simulink library "Gait_Selector"  (R2024a)
settings: Solver=VariableStepAuto  StartTime=0.0  StopTime=10.0  RelTol=1e-3
undefined symbols (not defined in the file): Length_torso, sampleTime, transferFunVal, Width_torso
libraries: simulink_extras x12, stand_still_Gait x1, trot_Gait x1, turn_left_Gait x1, turn_right_Gait x1, walk_back_Gait x1, walk_Gait x1, walk_left_Gait x1, walk_right_Gait x1
(part 2 of 2)

== system Gait_Selector/Gait Selector/Trot Gait - Drive Function/right Back Hip gait/If Action Subsystem ==
  In1 : Inport
  tdur : Inport  Port=2
  Add : Sum  Inputs=+-
  Constant : Constant  Value=1.5 * pi
  Divide : Product  Inputs=*/
  Gain1 : Gain  Gain=2/3
  Gain4 : Gain  Gain=2*pi
  Sin : Trigonometry
  Out1 : Outport
  wires:
  In1/1 -> Gain4/1
  Constant/1 -> Add/2
  Add/1 -> Gain1/1
  Gain1/1 -> Sin/1
  Sin/1 -> Out1/1
  Gain4/1 -> Divide/1
  tdur/1 -> Divide/2
  Divide/1 -> Add/1

== system Gait_Selector/Gait Selector/Trot Gait - Drive Function/right Back Hip gait/If Action Subsystem1 ==
  In1 : Inport
  tdur : Inport  Port=2
  Add : Sum  Inputs=+-
  Constant : Constant  Value=1.0 * pi
  Divide : Product  Inputs=*/
  Gain1 : Gain  Gain=2
  Gain4 : Gain  Gain=2*pi
  Sin : Trigonometry
  Out1 : Outport
  wires:
  Sin/1 -> Out1/1
  In1/1 -> Gain4/1
  Add/1 -> Gain1/1
  Constant/1 -> Add/2
  Gain1/1 -> Sin/1
  Gain4/1 -> Divide/1
  Divide/1 -> Add/1
  tdur/1 -> Divide/2

== system Gait_Selector/Gait Selector/Trot Gait - Drive Function/right Back Hip gait/If Action Subsystem2 ==
  In1 : Inport
  tdur : Inport  Port=2
  Add : Sum  Inputs=+-
  Constant : Constant  Value=1.25 * pi
  Divide : Product  Inputs=*/
  Gain1 : Gain  Gain=2/3
  Gain4 : Gain  Gain=2*pi
  Sin : Trigonometry  Operator=cos
  Out1 : Outport
  wires:
  Sin/1 -> Out1/1
  In1/1 -> Gain4/1
  Add/1 -> Gain1/1
  Constant/1 -> Add/2
  Gain1/1 -> Sin/1
  Gain4/1 -> Divide/1
  Divide/1 -> Add/1
  tdur/1 -> Divide/2

== system Gait_Selector/Gait Selector/Trot Gait - Drive Function/right Back Knee gait/If Action Subsystem4 ==
  In1 : Inport
  tdur : Inport  Port=2
  Add : Sum  Inputs=+-
  Constant : Constant  Value=0.75 * pi
  Divide : Product  Inputs=*/
  Gain1 : Gain  Gain=2
  Gain4 : Gain  Gain=2*pi
  Sin : Trigonometry
  Out1 : Outport
  wires:
  Sin/1 -> Out1/1
  In1/1 -> Gain4/1
  Add/1 -> Gain1/1
  Constant/1 -> Add/2
  Gain1/1 -> Sin/1
  Divide/1 -> Add/1
  Gain4/1 -> Divide/1
  tdur/1 -> Divide/2

== system Gait_Selector/Gait Selector/Trot Gait - Drive Function/right Front Hip gait/If Action Subsystem ==
  In1 : Inport
  tdur : Inport  Port=2
  Add : Sum  Inputs=+-
  Constant : Constant  Value=1.5 * pi
  Divide : Product  Inputs=*/
  Gain1 : Gain  Gain=2/3
  Gain4 : Gain  Gain=2*pi
  Sin : Trigonometry
  Out1 : Outport
  wires:
  In1/1 -> Gain4/1
  Constant/1 -> Add/2
  Add/1 -> Gain1/1
  Gain1/1 -> Sin/1
  Sin/1 -> Out1/1
  Gain4/1 -> Divide/1
  tdur/1 -> Divide/2
  Divide/1 -> Add/1

== system Gait_Selector/Gait Selector/Trot Gait - Drive Function/right Front Hip gait/If Action Subsystem1 ==
  In1 : Inport
  tdur : Inport  Port=2
  Add : Sum  Inputs=+-
  Constant : Constant  Value=1.0 * pi
  Divide : Product  Inputs=*/
  Gain1 : Gain  Gain=2
  Gain4 : Gain  Gain=2*pi
  Sin : Trigonometry
  Out1 : Outport
  wires:
  Sin/1 -> Out1/1
  In1/1 -> Gain4/1
  Add/1 -> Gain1/1
  Constant/1 -> Add/2
  Gain1/1 -> Sin/1
  Gain4/1 -> Divide/1
  Divide/1 -> Add/1
  tdur/1 -> Divide/2

== system Gait_Selector/Gait Selector/Trot Gait - Drive Function/right Front Hip gait/If Action Subsystem2 ==
  In1 : Inport
  tdur : Inport  Port=2
  Add : Sum  Inputs=+-
  Constant : Constant  Value=1.25 * pi
  Divide : Product  Inputs=*/
  Gain1 : Gain  Gain=2/3
  Gain4 : Gain  Gain=2*pi
  Sin : Trigonometry  Operator=cos
  Out1 : Outport
  wires:
  Sin/1 -> Out1/1
  In1/1 -> Gain4/1
  Add/1 -> Gain1/1
  Constant/1 -> Add/2
  Gain1/1 -> Sin/1
  Gain4/1 -> Divide/1
  Divide/1 -> Add/1
  tdur/1 -> Divide/2

== system Gait_Selector/Gait Selector/Trot Gait - Drive Function/right Front Knee gait/If Action Subsystem4 ==
  In1 : Inport
  tdur : Inport  Port=2
  Add : Sum  Inputs=+-
  Constant : Constant  Value=0.75 * pi
  Divide : Product  Inputs=*/
  Gain1 : Gain  Gain=2
  Gain4 : Gain  Gain=2*pi
  Sin : Trigonometry
  Out1 : Outport
  wires:
  Sin/1 -> Out1/1
  In1/1 -> Gain4/1
  Add/1 -> Gain1/1
  Constant/1 -> Add/2
  Gain1/1 -> Sin/1
  Divide/1 -> Add/1
  Gain4/1 -> Divide/1
  tdur/1 -> Divide/2

== system Gait_Selector/Gait Selector/Walk Gait - Drive Function/left Back Hip gait/If Action Subsystem ==
  In1 : Inport
  tdur : Inport  Port=2
  Add : Sum  Inputs=+-
  Constant : Constant  Value=1.5 * pi
  Divide : Product  Inputs=*/
  Gain1 : Gain  Gain=2/3
  Gain4 : Gain  Gain=2*pi
  Sin : Trigonometry
  Out1 : Outport
  wires:
  In1/1 -> Gain4/1
  Constant/1 -> Add/2
  Add/1 -> Gain1/1
  Gain1/1 -> Sin/1
  Sin/1 -> Out1/1
  Gain4/1 -> Divide/1
  tdur/1 -> Divide/2
  Divide/1 -> Add/1

== system Gait_Selector/Gait Selector/Walk Gait - Drive Function/left Back Hip gait/If Action Subsystem1 ==
  In1 : Inport
  tdur : Inport  Port=2
  Add : Sum  Inputs=+-
  Constant : Constant  Value=1.0 * pi
  Divide : Product  Inputs=*/
  Gain1 : Gain  Gain=2
  Gain4 : Gain  Gain=2*pi
  Sin : Trigonometry
  Out1 : Outport
  wires:
  Sin/1 -> Out1/1
  In1/1 -> Gain4/1
  Add/1 -> Gain1/1
  Constant/1 -> Add/2
  Gain1/1 -> Sin/1
  Gain4/1 -> Divide/1
  Divide/1 -> Add/1
  tdur/1 -> Divide/2

== system Gait_Selector/Gait Selector/Walk Gait - Drive Function/left Back Hip gait/If Action Subsystem2 ==
  In1 : Inport
  tdur : Inport  Port=2
  Add : Sum  Inputs=+-
  Constant : Constant  Value=1.25 * pi
  Divide : Product  Inputs=*/
  Gain1 : Gain  Gain=2/3
  Gain4 : Gain  Gain=2*pi
  Sin : Trigonometry  Operator=cos
  Out1 : Outport
  wires:
  Sin/1 -> Out1/1
  In1/1 -> Gain4/1
  Add/1 -> Gain1/1
  Constant/1 -> Add/2
  Gain1/1 -> Sin/1
  Gain4/1 -> Divide/1
  Divide/1 -> Add/1
  tdur/1 -> Divide/2

== system Gait_Selector/Gait Selector/Walk Gait - Drive Function/left Back Knee gait/If Action Subsystem4 ==
  In1 : Inport
  tdur : Inport  Port=2
  Add : Sum  Inputs=+-
  Constant : Constant  Value=0.75 * pi
  Divide : Product  Inputs=*/
  Gain1 : Gain  Gain=2
  Gain4 : Gain  Gain=2*pi
  Sin : Trigonometry
  Out1 : Outport
  wires:
  Sin/1 -> Out1/1
  In1/1 -> Gain4/1
  Add/1 -> Gain1/1
  Constant/1 -> Add/2
  Gain1/1 -> Sin/1
  Divide/1 -> Add/1
  Gain4/1 -> Divide/1
  tdur/1 -> Divide/2

== system Gait_Selector/Gait Selector/Walk Gait - Drive Function/left Fornt Knee gait/If Action Subsystem4 ==
  In1 : Inport
  tdur : Inport  Port=2
  Add : Sum  Inputs=+-
  Constant : Constant  Value=0.75 * pi
  Divide : Product  Inputs=*/
  Gain1 : Gain  Gain=2
  Gain4 : Gain  Gain=2*pi
  Sin : Trigonometry
  Out1 : Outport
  wires:
  Sin/1 -> Out1/1
  In1/1 -> Gain4/1
  Add/1 -> Gain1/1
  Constant/1 -> Add/2
  Gain1/1 -> Sin/1
  Divide/1 -> Add/1
  Gain4/1 -> Divide/1
  tdur/1 -> Divide/2

== system Gait_Selector/Gait Selector/Walk Gait - Drive Function/left Front Hip gait/If Action Subsystem ==
  In1 : Inport
  tdur : Inport  Port=2
  Add : Sum  Inputs=+-
  Constant : Constant  Value=1.5 * pi
  Divide : Product  Inputs=*/
  Gain1 : Gain  Gain=2/3
  Gain4 : Gain  Gain=2*pi
  Sin : Trigonometry
  Out1 : Outport
  wires:
  In1/1 -> Gain4/1
  Constant/1 -> Add/2
  Add/1 -> Gain1/1
  Gain1/1 -> Sin/1
  Sin/1 -> Out1/1
  Gain4/1 -> Divide/1
  tdur/1 -> Divide/2
  Divide/1 -> Add/1

== system Gait_Selector/Gait Selector/Walk Gait - Drive Function/left Front Hip gait/If Action Subsystem1 ==
  In1 : Inport
  tdur : Inport  Port=2
  Add : Sum  Inputs=+-
  Constant : Constant  Value=1.0 * pi
  Divide : Product  Inputs=*/
  Gain1 : Gain  Gain=2
  Gain4 : Gain  Gain=2*pi
  Sin : Trigonometry
  Out1 : Outport
  wires:
  Sin/1 -> Out1/1
  In1/1 -> Gain4/1
  Add/1 -> Gain1/1
  Constant/1 -> Add/2
  Gain1/1 -> Sin/1
  Gain4/1 -> Divide/1
  Divide/1 -> Add/1
  tdur/1 -> Divide/2

== system Gait_Selector/Gait Selector/Walk Gait - Drive Function/left Front Hip gait/If Action Subsystem2 ==
  In1 : Inport
  tdur : Inport  Port=2
  Add : Sum  Inputs=+-
  Constant : Constant  Value=1.25 * pi
  Divide : Product  Inputs=*/
  Gain1 : Gain  Gain=2/3
  Gain4 : Gain  Gain=2*pi
  Sin : Trigonometry  Operator=cos
  Out1 : Outport
  wires:
  Sin/1 -> Out1/1
  In1/1 -> Gain4/1
  Add/1 -> Gain1/1
  Constant/1 -> Add/2
  Gain1/1 -> Sin/1
  Gain4/1 -> Divide/1
  Divide/1 -> Add/1
  tdur/1 -> Divide/2

== system Gait_Selector/Gait Selector/Walk Gait - Drive Function/right Back Hip gait/If Action Subsystem ==
  In1 : Inport
  tdur : Inport  Port=2
  Add : Sum  Inputs=+-
  Constant : Constant  Value=1.5 * pi
  Divide : Product  Inputs=*/
  Gain1 : Gain  Gain=2/3
  Gain4 : Gain  Gain=2*pi
  Sin : Trigonometry
  Out1 : Outport
  wires:
  In1/1 -> Gain4/1
  Constant/1 -> Add/2
  Add/1 -> Gain1/1
  Gain1/1 -> Sin/1
  Sin/1 -> Out1/1
  Gain4/1 -> Divide/1
  tdur/1 -> Divide/2
  Divide/1 -> Add/1

== system Gait_Selector/Gait Selector/Walk Gait - Drive Function/right Back Hip gait/If Action Subsystem1 ==
  In1 : Inport
  tdur : Inport  Port=2
  Add : Sum  Inputs=+-
  Constant : Constant  Value=1.0 * pi
  Divide : Product  Inputs=*/
  Gain1 : Gain  Gain=2
  Gain4 : Gain  Gain=2*pi
  Sin : Trigonometry
  Out1 : Outport
  wires:
  Sin/1 -> Out1/1
  In1/1 -> Gain4/1
  Add/1 -> Gain1/1
  Constant/1 -> Add/2
  Gain1/1 -> Sin/1
  Gain4/1 -> Divide/1
  Divide/1 -> Add/1
  tdur/1 -> Divide/2

== system Gait_Selector/Gait Selector/Walk Gait - Drive Function/right Back Hip gait/If Action Subsystem2 ==
  In1 : Inport
  tdur : Inport  Port=2
  Add : Sum  Inputs=+-
  Constant : Constant  Value=1.25 * pi
  Divide : Product  Inputs=*/
  Gain1 : Gain  Gain=2/3
  Gain4 : Gain  Gain=2*pi
  Sin : Trigonometry  Operator=cos
  Out1 : Outport
  wires:
  Sin/1 -> Out1/1
  In1/1 -> Gain4/1
  Add/1 -> Gain1/1
  Constant/1 -> Add/2
  Gain1/1 -> Sin/1
  Gain4/1 -> Divide/1
  Divide/1 -> Add/1
  tdur/1 -> Divide/2

== system Gait_Selector/Gait Selector/Walk Gait - Drive Function/right Back Knee gait/If Action Subsystem4 ==
  In1 : Inport
  tdur : Inport  Port=2
  Add : Sum  Inputs=+-
  Constant : Constant  Value=0.75 * pi
  Divide : Product  Inputs=*/
  Gain1 : Gain  Gain=2
  Gain4 : Gain  Gain=2*pi
  Sin : Trigonometry
  Out1 : Outport
  wires:
  Sin/1 -> Out1/1
  In1/1 -> Gain4/1
  Add/1 -> Gain1/1
  Constant/1 -> Add/2
  Gain1/1 -> Sin/1
  Divide/1 -> Add/1
  Gain4/1 -> Divide/1
  tdur/1 -> Divide/2

== system Gait_Selector/Gait Selector/Walk Gait - Drive Function/right Front Hip gait/If Action Subsystem ==
  In1 : Inport
  tdur : Inport  Port=2
  Add : Sum  Inputs=+-
  Constant : Constant  Value=1.5 * pi
  Divide : Product  Inputs=*/
  Gain1 : Gain  Gain=2/3
  Gain4 : Gain  Gain=2*pi
  Sin : Trigonometry
  Out1 : Outport
  wires:
  In1/1 -> Gain4/1
  Constant/1 -> Add/2
  Add/1 -> Gain1/1
  Gain1/1 -> Sin/1
  Sin/1 -> Out1/1
  Gain4/1 -> Divide/1
  tdur/1 -> Divide/2
  Divide/1 -> Add/1

== system Gait_Selector/Gait Selector/Walk Gait - Drive Function/right Front Hip gait/If Action Subsystem1 ==
  In1 : Inport
  tdur : Inport  Port=2
  Add : Sum  Inputs=+-
  Constant : Constant  Value=1.0 * pi
  Divide : Product  Inputs=*/
  Gain1 : Gain  Gain=2
  Gain4 : Gain  Gain=2*pi
  Sin : Trigonometry
  Out1 : Outport
  wires:
  Sin/1 -> Out1/1
  In1/1 -> Gain4/1
  Add/1 -> Gain1/1
  Constant/1 -> Add/2
  Gain1/1 -> Sin/1
  Gain4/1 -> Divide/1
  Divide/1 -> Add/1
  tdur/1 -> Divide/2

== system Gait_Selector/Gait Selector/Walk Gait - Drive Function/right Front Hip gait/If Action Subsystem2 ==
  In1 : Inport
  tdur : Inport  Port=2
  Add : Sum  Inputs=+-
  Constant : Constant  Value=1.25 * pi
  Divide : Product  Inputs=*/
  Gain1 : Gain  Gain=2/3
  Gain4 : Gain  Gain=2*pi
  Sin : Trigonometry  Operator=cos
  Out1 : Outport
  wires:
  Sin/1 -> Out1/1
  In1/1 -> Gain4/1
  Add/1 -> Gain1/1
  Constant/1 -> Add/2
  Gain1/1 -> Sin/1
  Gain4/1 -> Divide/1
  Divide/1 -> Add/1
  tdur/1 -> Divide/2

== system Gait_Selector/Gait Selector/Walk Gait - Drive Function/right Front Knee gait/If Action Subsystem4 ==
  In1 : Inport
  tdur : Inport  Port=2
  Add : Sum  Inputs=+-
  Constant : Constant  Value=0.75 * pi
  Divide : Product  Inputs=*/
  Gain1 : Gain  Gain=2
  Gain4 : Gain  Gain=2*pi
  Sin : Trigonometry
  Out1 : Outport
  wires:
  Sin/1 -> Out1/1
  In1/1 -> Gain4/1
  Add/1 -> Gain1/1
  Constant/1 -> Add/2
  Gain1/1 -> Sin/1
  Divide/1 -> Add/1
  Gain4/1 -> Divide/1
  tdur/1 -> Divide/2

== matlab function Gait_Selector/Gait Selector/Balance Controler/MATLAB Function ==
  data: f_FL input; P0x output; P0y output; f_FR input; f_BL input; f_BR input; P0x_prev input; P0y_prev input; P0z_prev input; P1x_prev input; P1y_prev input; P1z_prev input; P2x_prev input; P2y_prev input; P2z_prev input; P3x_prev input; P3y_prev input; P3z_prev input; P0z output; P1x output; P1y output; P1z output; P2x output; P2y output; P2z output; P3x output; P3y output; P3z output; l_Torso input; w_Torso input; stabilize input
function [P0x,P0y,P0z,P1x,P1y,P1z,P2x,P2y,P2z,P3x,P3y,P3z] = ...
    balanceFunction(f_FL, f_FR, f_BL, f_BR,P0x_prev,P0y_prev,P0z_prev, ...
    P1x_prev,P1y_prev,P1z_prev,P2x_prev,P2y_prev,P2z_prev,P3x_prev, ...
    P3y_prev,P3z_prev,l_Torso, w_Torso, stabilize)

if f_FL * f_FR * f_BL * f_BR * stabilize == 0
    P0x = P0x_prev;
    P0y = P0y_prev;
    P0z = P0z_prev;
    P1x = P1x_prev;
    P1y = P1y_prev;
    P1z = P1z_prev;
    P2x = P2x_prev;
    P2y = P2y_prev;
    P2z = P2z_prev;
    P3x = P3x_prev;
    P3y = P3y_prev;
    P3z = P3z_prev;
else
    f_F= f_FL + f_FR;
    f_B= f_BL + f_BR;
    f_Total = f_F + f_B;
    dispX = -1 * l_Torso * (f_Total/2 - f_F) / f_Total * 0.2;

    f_L = f_FL + f_BL;
    f_R = f_FR + f_BR;
    dispY = -1 * w_Torso * (f_Total/2 - f_L) / f_Total * 0.2; 
    P0x = P0x_prev + dispX;
    P0y = P0y_prev + dispY;
    P0z = P0z_prev;
    P1x = P1x_prev + dispX;
    P1y = P1y_prev + dispY;
    P1z = P1z_prev;
    P2x = P2x_prev + dispX;
    P2y = P2y_prev + dispY;
    P2z = P2z_prev;
    P3x = P3x_prev + dispX;
    P3y = P3y_prev + dispY;
    P3z = P3z_prev;
    
end

== matlab function Gait_Selector/Gait Selector/Triggered Subsystem/MATLAB Function ==
  data: u input; activationTime output
function activationTime = getActivationTime(u)
    persistent t_start
    if isempty(t_start)
        t_start = u;
    end
    activationTime = t_start;
end

== matlab function Gait_Selector/Gait Selector/MATLAB Function ==
  data: c_old input; c_new input; t input; C_out output; t_change input; tdur_old input; tdur_new input; tdur_out output
function [C_out, tdur_out]= control_change(c_old, c_new, t, t_change, tdur_old, tdur_new)

time_since_change = t-t_change;
if c_old == 0 || t < tdur_old
    C_out = c_new;
    tdur_out = tdur_new;

else
    if time_since_change < tdur_old
        C_out = c_old;
        tdur_out = tdur_old;
    else
        if time_since_change < (tdur_old+0.01)
            C_out = 0;
            tdur_out = 0.01;
        else
            C_out = c_new;
            tdur_out = tdur_new;
        end
    end

end
end
